simulink model "DAAEncounter"  (R2018b)
settings: Solver=ode45  StartTime=0.0  StopTime=180  RelTol=1e-3  EnableMultiTasking=on
values from neighbouring files (symbols this model uses):
  enableHorzMan = 1    [DAAEncounterClass.m]
  enableVertMan = 0    [DAAEncounterClass.m]
  eventFileNames = {'event1'; 'event2'}    [DAAEncounterClass.m]
  ignorePrevAlert = 1    [DAAEncounterClass.m]
  sim_sampleTime = 0.1    [DAAEncounterClass.m]
undefined symbols (not defined in the file or in its folder): daa_turnRate_dps, daa_vertRate_fpm, dh_flag, dh_ftps, dpsi_flag, dpsi_radps, uasPilot_altitudeK, uasPilot_altitudeOffset, uasPilot_altitudeTheta, uasPilot_coordDelayK, uasPilot_coordDelayMin, uasPilot_coordDelayTheta, uasPilot_desiredTurnRate_dps, uasPilot_desiredVertRate_ftpm, uasPilot_deterministicMode, uasPilot_dt_s, uasPilot_executionDelayMin, uasPilot_executionDelayMu, uasPilot_initialDelayMin, uasPilot_initialDelayMu, uasPilot_maxRelativeHdg, uasPilot_meanUpdateTimes, uasPilot_mentalFilter_climbThresh_fps, uasPilot_mentalFilter_numSamp, uasPilot_mentalFilter_turnThresh_rad, uasPilot_minUpdateTimes, uasPilot_operatorEnabled, uasPilot_probDescend, uasPilot_probFollowMinDev, uasPilot_probLeftTurn, uasPilot_probTurn, uasPilot_reducedClimbAlt_ft, uasPilot_reducedTurnAngle_deg, uasPilot_seedChoose, uasPilot_seedCoordDelay, uasPilot_seedExecutionDelay, uasPilot_seedInitialDelay, uasPilot_seedTurn, uasPilot_seedUpdate, uasPilot_seedVertical, uasPilot_triggerLevel, uasPilot_turnK, uasPilot_turnOffset, uasPilot_turnTheta
libraries: simulink x4, BasicAircraftDynamicsBlock x3, FlattenAircraftEstimateBus x2, PerfectSurveillanceBlock x2, DaidalusV201Block x1, HysteresisFilterBlock x1, MofNFilterBlock x1, CommonMetricsBlock x1, SLoWCBlock x1, WellClearMetricsBlock x1, NullAircraftEstimateBus x1, uas_pilot_model_r6 x1
(part 2 of 2)

== system DAAEncounter/Ownship Dynamics and Trajectory/Nominal Commands and Trajectory ==
  AC1 - Basic Aircraft Dynamics : BasicAircraftDynamicsBlock/Basic Aircraft Dynamics  ts_dynamics=.1  v_ftps_0=ac1dyn_v_ftps  N_ft_0=ac1dyn_N_ft  E_ft_0=ac1dyn_E_ft  h_ft_0=ac1dyn_h_ft  psi_rad_0=ac1dyn_psi_rad  theta_rad_0=ac1dyn_theta_rad  phi_rad_0=ac1dyn_phi_rad  a_ftpss_0=ac1dyn_a_ftpss  v_ftps_max=ac1dyn_con.maxAirspeed_ftps  v_ftps_min=ac1dyn_con.minAirspeed_ftps  dv_ftpss_max=ac1dyn_con.maxAcceleration_ftpss  dv_ftpss_min=ac1dyn_con.minAcceleration_ftpss  dh_ftps_max=ac1dyn_con.maxVerticalRate_ftps  dh_ftps_min=ac1dyn_con.minVerticalRate_ftps  q_radps_max=ac1dyn_con.maxPitchRate_radps  phi_rad_max=ac1dyn_con.maxBankAngle_rad  dphi_radps_max=ac1dyn_con.maxRollRate_radps  r_radps_max=ac1dyn_con.maxYawRate_radps  pNUM=ac1dyn_con.dynamicsNumeratorRollRate  pDEN=ac1dyn_con.dynamicsDenominatorRollRate  hNUM=ac1dyn_con.dynamicsNumeratorVerticalRate  hDEN=ac1dyn_con.dynamicsDenominatorVerticalRate  rNUM=ac1dyn_con.dynamicsNumeratorYawRate  rDEN=ac1dyn_con.dynamicsDenominatorYawRate  lat0_rad=ac2dyn_lat0_rad  lon0_rad=ac2dyn_lon0_rad  alt_ft=ac2dyn_alt0_ft
  AC1 - Nominal Trajectory : Subsystem  AncestorBlock=NominalTrajectory/Nominal Trajectory  mask(Logic and Response: Nominal Trajectory){eventFilename=eventFileNames{1}, ts=.1}
      mask prompts: eventFilename "Event matrix mat filename"; ts "Dynamic Update Rate"
      mask help:
      | The "Nominal Trajectory" Logic and Response Block describes the nominal
      | trajectory of an aircraft as defined in a "event matrix" typically sampled
      | from the encounter model.
      |
      | Logic and Response: Nominal Trajectory loads aircaft motion
      | commands from a MATLAB MAT file containing an event matrix of climb rates,
      | turn rates, and longitudinal accelerations, and presents them as a
      | CASSATT v6 AircraftCommands bus.
      |
      | The specified MAT file must contain a single matrix variable with four
      | rows.  The rows are
      |   - Time of control value change in seconds
      |   - Climb rate in feet per second
      |   - Turn rate in radians per second
      |   - Longitudinal acceleration in feet per second squared
      |
      | These control quantities (climb rate, turn rate acceleration) are assumed
      | remain constant between the times specified in the event matrix (zero order
      | hold).  The first / last control values in the event matrix are assumed to
      | preexist / persist at the value infinitely backwards / forwards in time.
      mask init:
      | set_param( [ gcb '/FromFile' ], 'Filename', eventFilename )
      mask Help:
      | The "Nominal Trajectory" Logic and Response Block describes the nominal
      | trajectory of an aircraft as defined in a "event matrix" typically sampled
      | from the encounter model.
      | 
      | Logic and Response: Nominal Trajectory loads aircaft motion
      | commands from a MATLAB MAT file containing an event matrix of climb rates,
      | turn rates, and longitudinal accelerations, and presents them as a
      | CASSATT v6 AircraftCommands bus.
      | 
      | The specified MAT file must contain a single matrix variable with four
      | rows.  The rows are
      |   - Time of control value change in seconds
      |   - Climb rate in feet per second
      |   - Turn rate in radians per second
      |   - Longitudinal acceleration in feet per second squared
      | 
      | These control quantities (climb rate, turn rate acceleration) are assumed
      | remain constant between the times specified in the event matrix (zero order
      | hold).  The first / last control values in the event matrix are assumed to
      | preexist / persist at the value infinitely backwards / forwards in time.
      | 
      | CASSATT v6 Aircraft dynamics blocks, which calculate the positions and velocities
      | traced out by an aircraft's trajectory,
      | require input signals specifying controls for the aircraft (e.g. turn rate, acceleration, climb rate)
      | in the form of a AircraftCommands bus.
      | This block allows the user to specify what these controls in a Matlab MAT file.
      | Include this in your simulation to describe the nominal motion of an aircraft
      | trajectory you have sampled from the Lincoln Encounter Models.
  Terminator : Terminator
  Nominal Commands : Outport
  NominalOwnshipState : Outport  Port=2
  NominalOwnshipStateRate : Outport  Port=3
  wires:
  AC1 - Nominal Trajectory/1(Aircraft Commands) -> AC1 - Basic Aircraft Dynamics/1, Nominal Commands/1
  AC1 - Basic Aircraft Dynamics/1 -> NominalOwnshipState/1  "Aircraft1"
  AC1 - Basic Aircraft Dynamics/2 -> Terminator/1
  AC1 - Basic Aircraft Dynamics/3 -> NominalOwnshipStateRate/1

== system DAAEncounter/Pilot/Format Maneuver As AircraftCommand ==
  Maneuver Flag : Inport  OutDataTypeStr=boolean
  Hrz Maneuver : Inport  Port=2
  Vrt Maneuver : Inport  Port=3
  Nominal Cmd : Inport  Port=4  OutDataTypeStr=Bus: AircraftCommands
  Own State : Inport  Port=5  OutDataTypeStr=Bus: AircraftState
  UAS Nominal Traj : Inport  Port=6
  Get Previous Command : Subsystem
  Horizontal Maneuver : Subsystem  TreatAsAtomicUnit=on
  Unit Delay : UnitDelay  SampleTime=-1
  Vertical Maneuver : Subsystem  TreatAsAtomicUnit=on
  Command Out : Outport  OutDataTypeStr=Bus: AircraftCommands
  wires:
  Maneuver Flag/1 -> Vertical Maneuver/4(Maneuver Flag), Horizontal Maneuver/4(Maneuver Flag), Get Previous Command/3(Maneuver Flag)
  Nominal Cmd/1 -> Get Previous Command/2(Nominal Cmd)
  Unit Delay/1 -> Get Previous Command/1(Cmd In)
  Own State/1 -> Vertical Maneuver/3(Own State), Horizontal Maneuver/3(Own State)
  Hrz Maneuver/1 -> Horizontal Maneuver/2(Maneuver)
  Vrt Maneuver/1 -> Vertical Maneuver/2(Maneuver)
  Horizontal Maneuver/1(Cmd Out) -> Vertical Maneuver/1(Command In)
  Vertical Maneuver/1(Cmd Out) -> Command Out/1, Unit Delay/1
  Get Previous Command/1(Cmd Out) -> Horizontal Maneuver/1(Command In)
  UAS Nominal Traj/1 -> Vertical Maneuver/5(UAS Nominal Traj)

== system DAAEncounter/Pilot/Horizontal and Vertical guidance enabler ==
  Unmodified Guidance : Inport
  " " : Constant  Value=enableVertMan
  " 1" : Constant  Value=enableHorzMan
  Horizontal Band manipulation : MATLAB Function  TreatAsAtomicUnit=on
  Switch : Switch  Criteria=u2 > Threshold
  Switch1 : Switch  Criteria=u2 > Threshold
  Vertical Band manipulation : MATLAB Function  TreatAsAtomicUnit=on
  Modified Guidance : Outport
  wires:
  " "/1 -> Switch/2
  Vertical Band manipulation/1(Guidance_out) -> Switch/3  "Guidance"
  Unmodified Guidance/1 -> Vertical Band manipulation/1(Guidance_in), Switch/1
  " 1"/1 -> Switch1/2
  Switch/1 -> Switch1/1, Horizontal Band manipulation/1(Guidance_in)
  Switch1/1 -> Modified Guidance/1
  Horizontal Band manipulation/1(Guidance_out) -> Switch1/3

== system DAAEncounter/Pilot/Subsystem ==
  Own State : Inport
  Alert Level : Inport  Port=2
  Trigger : Inport  Port=3
  Guidance : Inport  Port=4
  Max Turn Rt : Inport  Port=5
  Max Vert Rt : Inport  Port=6
  Enable : EnablePort
  Null AircraftEstimate Bus : NullAircraftEstimateBus/Null AircraftEstimate Bus
  UAS Pilot Model Release 6.1 : uas_pilot_model_r6/UAS Pilot Model Release 6.1  dt=dt  operator_enabled=operator_enabled  deterministicMode=deterministicMode  mean_initial_delay=mean_initial_delay  min_initial_delay=min_initial_delay  coord_delay_k=coord_delay_k  coord_delay_theta=coord_delay_theta  coord_delay_min=coord_delay_min  mean_exec_delay=mean_exec_delay  min_exec_delay=min_exec_delay  min_upd_times=min_upd_times  mean_upd_times=mean_upd_times  rng_seed_initial=rng_seed_initial  rng_seed_coord=rng_seed_coord  rng_seed_execution=rng_seed_execution  rng_seed_update=rng_seed_update  prob_follow_min=prob_follow_min  prob_turn_left=prob_turn_left  prob_turn_table=prob_turn  max_hdg_diff=max_hdg_diff  prob_descend=prob_descend  turn_k=turn_k  turn_theta=turn_theta  turn_offset=turn_offset  turn_k_alt=uasPilot_turnK_alt  turn_theta_alt=uasPilot_turnTheta_alt  turn_offset_alt=uasPilot_turnOffset_alt  alt_k=alt_k  alt_theta=alt_theta  alt_offset=alt_offset  rng_seed_horz=rng_seed_horz  rng_seed_vert=rng_seed_vert  rng_seed_horz_vs_vert=rng_seed_horz_vs_vert  mental_filter_samples=0  mental_filter_climb_thresh=0  mental_filter_turn_thresh=0
  Maneuver Flag : Outport
  Hrz Maneuver : Outport  Port=2
  Vrt Maneuver : Outport  Port=3
  wires:
  Own State/1 -> UAS Pilot Model Release 6.1/1
  Null AircraftEstimate Bus/1 -> UAS Pilot Model Release 6.1/2
  UAS Pilot Model Release 6.1/2 -> Hrz Maneuver/1
  Guidance/1 -> UAS Pilot Model Release 6.1/5
  Max Turn Rt/1 -> UAS Pilot Model Release 6.1/6
  Trigger/1 -> UAS Pilot Model Release 6.1/4
  Alert Level/1 -> UAS Pilot Model Release 6.1/3
  UAS Pilot Model Release 6.1/3 -> Vrt Maneuver/1
  UAS Pilot Model Release 6.1/1 -> Maneuver Flag/1
  Max Vert Rt/1 -> UAS Pilot Model Release 6.1/7

== system DAAEncounter/Pilot/Trigger ==
  Alert Level : Inport
  Filter Alerts : Subsystem  AncestorBlock=CABSAA_ModelLibrary/Filter Alerts  mask(Filter Alerts){trigger_level=trigger_level}
      mask prompts: trigger_level "Alert Level for Trigger"
      mask help: Holds alert level for at least the specified time unless the alert level increases.
  Trigger : Outport
  wires:
  Filter Alerts/1(Trigger) -> Trigger/1
  Alert Level/1 -> Filter Alerts/1(Alert Level In)

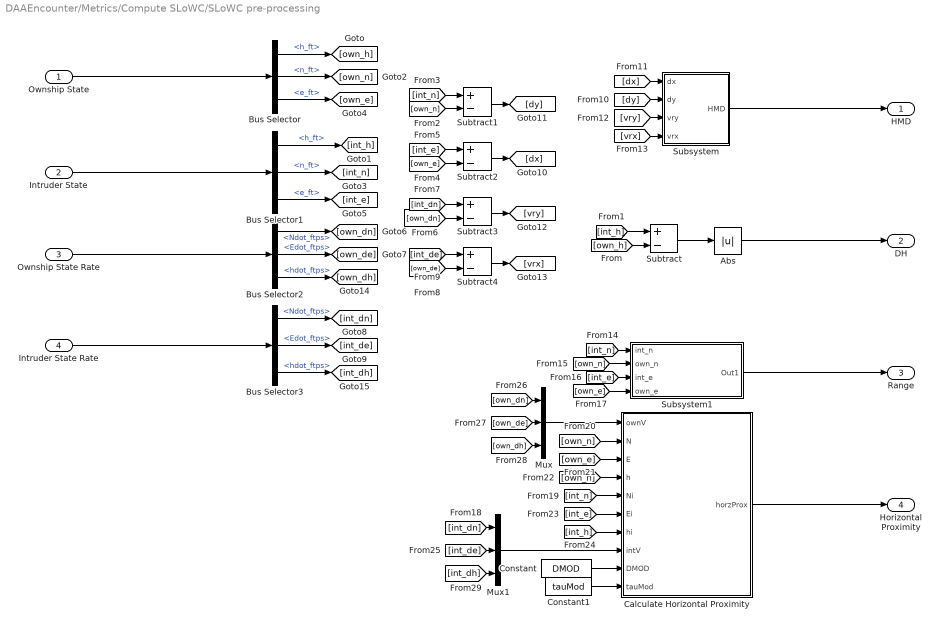
== system DAAEncounter/Metrics/Compute SLoWC/SLoWC pre-processing ==
  Ownship State : Inport
  Intruder State : Inport  Port=2
  Ownship State Rate : Inport  Port=3
  Intruder State Rate : Inport  Port=4
  Abs : Abs
  Bus Selector : BusSelector  OutputSignals=h_ft,n_ft,e_ft
  Bus Selector1 : BusSelector  OutputSignals=h_ft,n_ft,e_ft
  Bus Selector2 : BusSelector  OutputSignals=Ndot_ftps,Edot_ftps,hdot_ftps
  Bus Selector3 : BusSelector  OutputSignals=Ndot_ftps,Edot_ftps,hdot_ftps
  Calculate Horizontal Proximity : MATLAB Function  TreatAsAtomicUnit=on
  Constant : Constant  Value=DMOD
  Constant1 : Constant  Value=tauMod
  Mux : Mux  Inputs=3
  Mux1 : Mux  Inputs=3
  Subsystem : Subsystem
  Subsystem1 : Subsystem
  Subtract{,1..4} (5 alike) : Sum  Inputs=+-
  HMD : Outport
  DH : Outport  Port=2
  Range : Outport  Port=3
  Horizontal Proximity : Outport  Port=4
  wires:
  Subtract/1 -> Abs/1
  [own_dh] -> Mux/3
  Bus Selector/1 -> [own_h]  "<h_ft>"
  [own_dn] -> Subtract3/2
  Bus Selector1/3 -> [int_e]  "<e_ft>"
  [int_n] -> Calculate Horizontal Proximity/5(Ni)
  Bus Selector3/3 -> [int_dh]  "<hdot_ftps>"
  [int_h] -> Calculate Horizontal Proximity/7(hi)
  [int_e] -> Subtract2/1
  [own_h] -> Subtract/2
  Intruder State/1 -> Bus Selector1/1
  [own_n] -> Subtract1/2
  Constant/1 -> Calculate Horizontal Proximity/9(DMOD)
  [own_e] -> Subtract2/2
  [int_dh] -> Mux1/3
  Subtract4/1 -> [vrx]
  [int_h] -> Subtract/1
  Bus Selector1/1 -> [int_h]  "<h_ft>"
  [vry] -> Subsystem/3(vry)
  [own_n] -> Calculate Horizontal Proximity/2(N)
  Bus Selector3/1 -> [int_dn]  "<Ndot_ftps>"
  Subtract2/1 -> [dx]
  Bus Selector1/2 -> [int_n]  "<n_ft>"
  Bus Selector/2 -> [own_n]  "<n_ft>"
  Subtract3/1 -> [vry]
  [int_e] -> Subsystem1/3(int_e)
  [own_de] -> Mux/2
  Mux1/1 -> Calculate Horizontal Proximity/8(intV)
  Subtract1/1 -> [dy]
  [own_h] -> Calculate Horizontal Proximity/4(h)
  [dy] -> Subsystem/2(dy)
  [own_n] -> Subsystem1/2(own_n)
  [int_dn] -> Mux1/1
  Subsystem/1(HMD) -> HMD/1
  Bus Selector2/2 -> [own_de]  "<Edot_ftps>"
  [int_n] -> Subtract1/1
  Bus Selector2/3 -> [own_dh]  "<hdot_ftps>"
  [int_de] -> Subtract4/1
  Constant1/1 -> Calculate Horizontal Proximity/10(tauMod)
  Bus Selector/3 -> [own_e]  "<e_ft>"
  Subsystem1/1(Out1) -> Range/1
  [int_n] -> Subsystem1/1("int_n ")
  [int_e] -> Calculate Horizontal Proximity/6(Ei)
  [own_de] -> Subtract4/2
  Bus Selector3/2 -> [int_de]  "<Edot_ftps>"
  Mux/1 -> Calculate Horizontal Proximity/1(ownV)
  [dx] -> Subsystem/1("dx ")
  [int_dn] -> Subtract3/1
  Intruder State Rate/1 -> Bus Selector3/1
  [vrx] -> Subsystem/4(vrx)
  [own_dn] -> Mux/1
  Bus Selector2/1 -> [own_dn]  "<Ndot_ftps>"
  Abs/1 -> DH/1
  [own_e] -> Calculate Horizontal Proximity/3(E)
  Calculate Horizontal Proximity/1(horzProx) -> Horizontal Proximity/1
  Ownship State/1 -> Bus Selector/1
  [int_de] -> Mux1/2
  [own_e] -> Subsystem1/4(own_e)
  Ownship State Rate/1 -> Bus Selector2/1

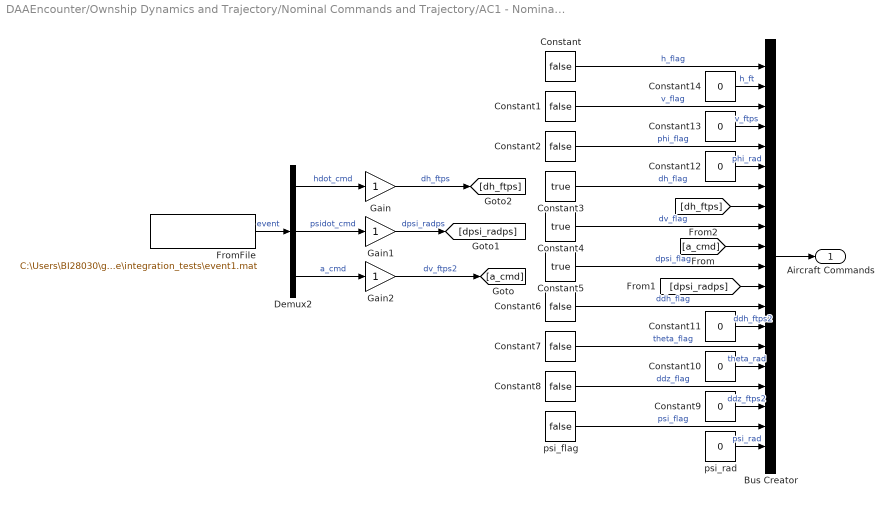
== system DAAEncounter/Ownship Dynamics and Trajectory/Nominal Commands and Trajectory/AC1 - Nominal Trajectory ==
  Bus Creator : BusCreator  Inputs=20  OutDataTypeStr=Bus: AircraftCommands  NonVirtualBus=on
  Constant{,1..2,6..8} (6 alike) : Constant  Value=false
  Constant{9..14} (6 alike) : Constant  Value=0
  Constant3 : Constant  Value=true
  Constant4 : Constant  Value=true
  Constant5 : Constant  Value=true
  Demux2 : Demux  Outputs=3
  FromFile : FromFile  FileName=C:\Users\BI28030\git_cln\DEGAS_cln\D_cln\CASSATT\code\integration_tests\event1.mat  SampleTime=ts  ExtrapolationBeforeFirstDataPoint=Hold first value  InterpolationWithinTimeRange=Zero order hold  ExtrapolationAfterLastDataPoint=Hold last value
  Gain : Gain
  Gain1 : Gain
  Gain2 : Gain
  psi_flag : Constant  Value=false
  psi_rad : Constant  Value=0
  Aircraft Commands : Outport  OutDataTypeStr=Bus: AircraftCommands
  wires:
  [dh_ftps] -> Bus Creator/8
  [dpsi_radps] -> Bus Creator/12
  [a_cmd] -> Bus Creator/10
  psi_rad/1 -> Bus Creator/20  "psi_rad"
  psi_flag/1 -> Bus Creator/19  "psi_flag"
  Demux2/1 -> Gain/1  "hdot_cmd"
  Demux2/2 -> Gain1/1  "psidot_cmd"
  Demux2/3 -> Gain2/1  "a_cmd"
  FromFile/1 -> Demux2/1  "event"
  Bus Creator/1 -> Aircraft Commands/1
  Constant/1 -> Bus Creator/1  "h_flag"
  Constant1/1 -> Bus Creator/3  "v_flag"
  Constant2/1 -> Bus Creator/5  "phi_flag"
  Constant3/1 -> Bus Creator/7  "dh_flag"
  Constant4/1 -> Bus Creator/9  "dv_flag"
  Constant5/1 -> Bus Creator/11  "dpsi_flag"
  Constant6/1 -> Bus Creator/13  "ddh_flag"
  Constant7/1 -> Bus Creator/15  "theta_flag"
  Constant8/1 -> Bus Creator/17  "ddz_flag"
  Gain/1 -> [dh_ftps]  "dh_ftps"
  Gain1/1 -> [dpsi_radps]  "dpsi_radps"
  Gain2/1 -> [a_cmd]  "dv_ftps2"
  Constant9/1 -> Bus Creator/18  "ddz_ftps2"
  Constant11/1 -> Bus Creator/14  "ddh_ftps2"
  Constant10/1 -> Bus Creator/16  "theta_rad"
  Constant14/1 -> Bus Creator/2  "h_ft"
  Constant13/1 -> Bus Creator/4  "v_ftps"
  Constant12/1 -> Bus Creator/6  "phi_rad"

== system DAAEncounter/Pilot/Format Maneuver As AircraftCommand/Get Previous Command ==
  Cmd In : Inport
  Nominal Cmd : Inport  Port=2
  Maneuver Flag : Inport  Port=3
  Data Type Conversion : DataTypeConversion  OutDataTypeStr=double
  Memory : Memory  InheritSampleTime=on
  Switch : Switch  Criteria=u2 > Threshold
  Cmd Out : Outport
  wires:
  Maneuver Flag/1 -> Memory/1
  Memory/1 -> Data Type Conversion/1
  Nominal Cmd/1 -> Switch/3
  Switch/1 -> Cmd Out/1
  Cmd In/1 -> Switch/1
  Data Type Conversion/1 -> Switch/2

== system DAAEncounter/Pilot/Format Maneuver As AircraftCommand/Horizontal Maneuver ==
  Command In : Inport
  Maneuver : Inport  Port=2
  Own State : Inport  Port=3
  Maneuver Flag : Inport  Port=4  OutDataTypeStr=boolean
  Bus Selector : BusSelector  OutputSignals=type
  Compare To Constant : simulink/Logic and Bit Operations/Compare To Constant  relop===  const=1  OutDataTypeStr=boolean
  Data Type Conversion1 : DataTypeConversion  OutDataTypeStr=double
  Logical Operator : Logic  AllPortsSameDT=off  OutDataTypeStr=boolean
  Set Desired Turn Rate : Subsystem
  Switch : Switch  Criteria=u2 > Threshold
  Cmd Out : Outport
  wires:
  Bus Selector/1 -> Compare To Constant/1  "<type>"
  Maneuver/1 -> Set Desired Turn Rate/2(Maneuver Magnitude), Bus Selector/1
  Own State/1 -> Set Desired Turn Rate/3(Own State)
  Maneuver Flag/1 -> Data Type Conversion1/1
  Logical Operator/1 -> Switch/2
  Command In/1 -> Switch/3, Set Desired Turn Rate/1(Cmd In)
  Data Type Conversion1/1 -> Logical Operator/1
  Compare To Constant/1 -> Logical Operator/2
  Set Desired Turn Rate/1(Cmd Out) -> Switch/1
  Switch/1 -> Cmd Out/1

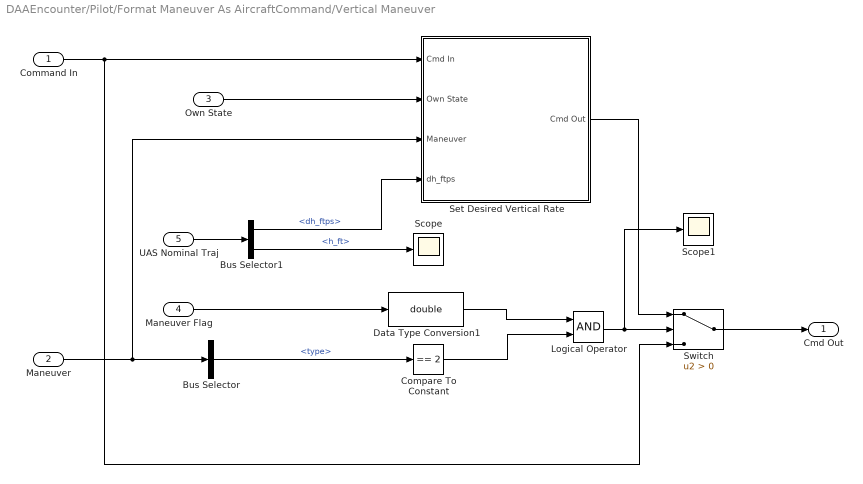
== system DAAEncounter/Pilot/Format Maneuver As AircraftCommand/Vertical Maneuver ==
  Command In : Inport
  Maneuver : Inport  Port=2
  Own State : Inport  Port=3
  Maneuver Flag : Inport  Port=4  OutDataTypeStr=boolean
  UAS Nominal Traj : Inport  Port=5
  Bus Selector1 : BusSelector  OutputSignals=dh_ftps,h_ft
  Bus Selector : BusSelector  OutputSignals=type
  Compare To Constant : simulink/Logic and Bit Operations/Compare To Constant  relop===  const=2  OutDataTypeStr=boolean
  Data Type Conversion1 : DataTypeConversion  OutDataTypeStr=double
  Logical Operator : Logic  AllPortsSameDT=off  OutDataTypeStr=boolean
  Scope : Scope
  Scope1 : Scope
  Set Desired Vertical Rate : Subsystem
  Switch : Switch  Criteria=u2 > Threshold
  Cmd Out : Outport
  wires:
  Bus Selector/1 -> Compare To Constant/1  "<type>"
  Maneuver Flag/1 -> Data Type Conversion1/1
  Switch/1 -> Cmd Out/1
  Data Type Conversion1/1 -> Logical Operator/1
  Compare To Constant/1 -> Logical Operator/2
  Command In/1 -> Set Desired Vertical Rate/1(Cmd In), Switch/3
  Set Desired Vertical Rate/1(Cmd Out) -> Switch/1
  UAS Nominal Traj/1 -> Bus Selector1/1
  Bus Selector1/2 -> Scope/1  "<h_ft>"
  Own State/1 -> Set Desired Vertical Rate/2(Own State)
  Maneuver/1 -> Set Desired Vertical Rate/3(Maneuver), Bus Selector/1
  Bus Selector1/1 -> Set Desired Vertical Rate/4(dh_ftps)  "<dh_ftps>"
  Logical Operator/1 -> Scope1/1, Switch/2

== system DAAEncounter/Pilot/Trigger/Filter Alerts ==
  Alert Level In : Inport
  Constant6 : Constant  Value=trigger_level
  Relational Operator : RelationalOperator  OutDataTypeStr=boolean  RndMeth=Nearest
  Trigger : Outport
  wires:
  Relational Operator/1 -> Trigger/1
  Constant6/1 -> Relational Operator/2
  Alert Level In/1 -> Relational Operator/1

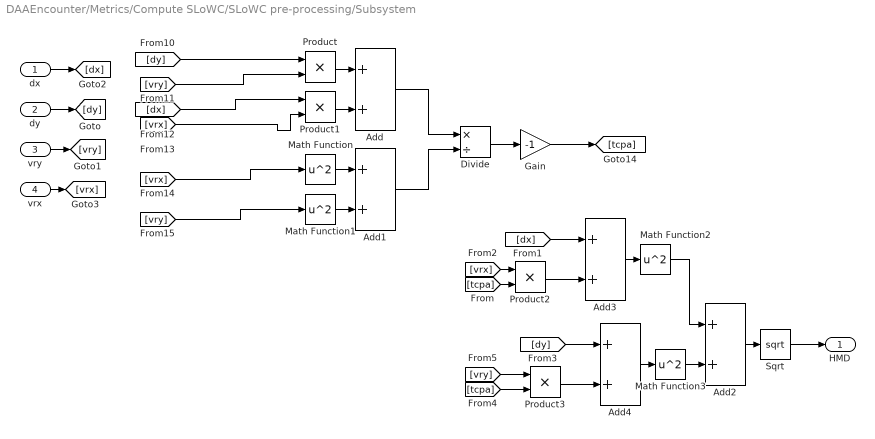
== system DAAEncounter/Metrics/Compute SLoWC/SLoWC pre-processing/Subsystem ==
  "dx " : Inport
  dy : Inport  Port=2
  vry : Inport  Port=3
  vrx : Inport  Port=4
  Add{,1..4} (5 alike) : Sum
  Divide : Product  Inputs=*/
  Gain : Gain  Gain=-1
  Math Function{,1..3} (4 alike) : Math  Operator=square  SaturateOnIntegerOverflow=on
  Product{,1..3} (4 alike) : Product
  Sqrt : Sqrt  SaturateOnIntegerOverflow=on
  HMD : Outport
  wires:
  Math Function1/1 -> Add1/2
  Gain/1 -> [tcpa]
  Add/1 -> Divide/1
  Math Function/1 -> Add1/1
  Product1/1 -> Add/2
  Product/1 -> Add/1
  [vrx] -> Math Function/1
  [vrx] -> Product1/2
  [dx] -> Product1/1
  Divide/1 -> Gain/1
  Add1/1 -> Divide/2
  [vry] -> Product/2
  [dy] -> Product/1
  [vry] -> Math Function1/1
  Sqrt/1 -> HMD/1
  Add2/1 -> Sqrt/1
  Math Function2/1 -> Add2/1
  Add3/1 -> Math Function2/1
  [dx] -> Add3/1
  [vrx] -> Product2/1
  Product2/1 -> Add3/2
  [tcpa] -> Product2/2
  Add4/1 -> Math Function3/1
  Math Function3/1 -> Add2/2
  Product3/1 -> Add4/2
  [dy] -> Add4/1
  [tcpa] -> Product3/2
  [vry] -> Product3/1
  "dx "/1 -> [dx]
  vrx/1 -> [vrx]
  vry/1 -> [vry]
  dy/1 -> [dy]

== system DAAEncounter/Metrics/Compute SLoWC/SLoWC pre-processing/Subsystem1 ==
  "int_n " : Inport
  own_n : Inport  Port=2
  int_e : Inport  Port=3
  own_e : Inport  Port=4
  Add1 : Sum
  Math Function : Math  Operator=square  SaturateOnIntegerOverflow=on
  Math Function1 : Math  Operator=square  SaturateOnIntegerOverflow=on
  Sqrt : Sqrt  SaturateOnIntegerOverflow=on
  Subtract5 : Sum  Inputs=+-
  Subtract6 : Sum  Inputs=+-
  Out1 : Outport
  wires:
  Math Function/1 -> Add1/1
  Add1/1 -> Sqrt/1
  Math Function1/1 -> Add1/2
  Subtract5/1 -> Math Function/1
  Sqrt/1 -> Out1/1
  Subtract6/1 -> Math Function1/1
  int_e/1 -> Subtract6/1
  own_n/1 -> Subtract5/2
  "int_n "/1 -> Subtract5/1
  own_e/1 -> Subtract6/2

== system DAAEncounter/Pilot/Format Maneuver As AircraftCommand/Horizontal Maneuver/Set Desired Turn Rate ==
  Cmd In : Inport
  Maneuver Magnitude : Inport  Port=2
  Own State : Inport  Port=3
  Bus Assignment1 : BusAssignment  AssignedSignals=dpsi_flag,dpsi_radps
  Constant : Constant  OutDataTypeStr=boolean
  Desired Heading to Turn Rate : Subsystem
  Cmd Out : Outport
  wires:
  Own State/1 -> Desired Heading to Turn Rate/2(Own State)
  Bus Assignment1/1 -> Cmd Out/1
  Cmd In/1 -> Bus Assignment1/1
  Constant/1 -> Bus Assignment1/2
  Maneuver Magnitude/1 -> Desired Heading to Turn Rate/1(Heading Cmd)
  Desired Heading to Turn Rate/1(Turn Rate) -> Bus Assignment1/3

== system DAAEncounter/Pilot/Format Maneuver As AircraftCommand/Vertical Maneuver/Set Desired Vertical Rate ==
  Cmd In : Inport
  Own State : Inport  Port=2
  Maneuver : Inport  Port=3
  dh_ftps : Inport  Port=4
  Bus Assignment : BusAssignment  AssignedSignals=dh_flag,dh_ftps
  Constant : Constant  OutDataTypeStr=boolean
  Constant1 : Constant  Value=enableVertMan
  Desired Altitude to Vertical Rate : Subsystem
  Multiport Switch : MultiPortSwitch  DataPortOrder=Specify indices  DataPortIndices={1 0}
  Scope : Scope
  Cmd Out : Outport
  wires:
  Bus Assignment/1 -> Cmd Out/1
  Own State/1 -> Desired Altitude to Vertical Rate/2(Own State)
  Cmd In/1 -> Bus Assignment/1
  Constant/1 -> Bus Assignment/2
  Maneuver/1 -> Desired Altitude to Vertical Rate/1(Altitude Cmd)
  dh_ftps/1 -> Multiport Switch/3
  Constant1/1 -> Multiport Switch/1
  Desired Altitude to Vertical Rate/1(Vert Rt) -> Scope/1, Multiport Switch/2
  Multiport Switch/1 -> Bus Assignment/3

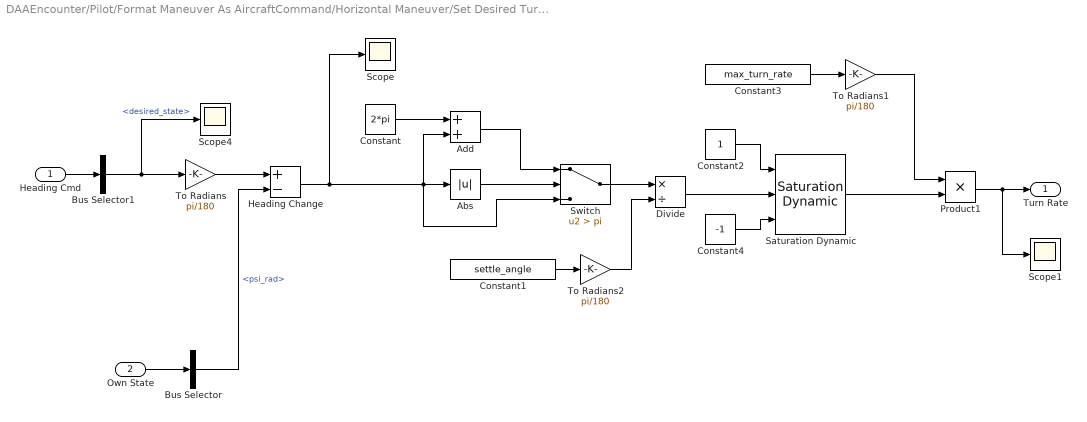
== system DAAEncounter/Pilot/Format Maneuver As AircraftCommand/Horizontal Maneuver/Set Desired Turn Rate/Desired Heading to Turn Rate ==
  Heading Cmd : Inport
  Own State : Inport  Port=2
  Abs : Abs
  Add : Sum
  Bus Selector : BusSelector  OutputSignals=psi_rad
  Bus Selector1 : BusSelector  OutputSignals=desired_state
  Constant : Constant  Value=2*pi
  Constant1 : Constant  Value=settle_angle
  Constant2 : Constant
  Constant3 : Constant  Value=max_turn_rate
  Constant4 : Constant  Value=-1
  Divide : Product  Inputs=*/
  Heading Change : Sum  Inputs=+-
  Product1 : Product  RndMeth=Zero
  Saturation Dynamic : simulink/Discontinuities/Saturation Dynamic  OutMin=[]  OutMax=[]  OutDataTypeStr=Inherit: Same as second input  OutDataType=fixdt(1, 16)  OutScaling=2^-10  DoSatur=off
  Scope : Scope
  Scope1 : Scope
  Scope4 : Scope
  Switch : Switch  Criteria=u2 > Threshold  Threshold=pi
  To Radians : Gain  Gain=pi/180
  To Radians1 : Gain  Gain=pi/180
  To Radians2 : Gain  Gain=pi/180
  Turn Rate : Outport
  wires:
  Constant/1 -> Add/1
  Switch/1 -> Divide/1
  Constant4/1 -> Saturation Dynamic/3
  Divide/1 -> Saturation Dynamic/2
  Abs/1 -> Switch/2
  Heading Change/1 -> Scope/1, Switch/3, Abs/1, Add/2
  Add/1 -> Switch/1
  Own State/1 -> Bus Selector/1
  Bus Selector/1 -> Heading Change/2  "<psi_rad>"
  To Radians/1 -> Heading Change/1
  Constant2/1 -> Saturation Dynamic/1
  Saturation Dynamic/1 -> Product1/2
  Constant1/1 -> To Radians2/1
  Product1/1 -> Scope1/1, Turn Rate/1
  Constant3/1 -> To Radians1/1
  To Radians1/1 -> Product1/1
  To Radians2/1 -> Divide/2
  Bus Selector1/1 -> To Radians/1, Scope4/1  "<desired_state>"
  Heading Cmd/1 -> Bus Selector1/1

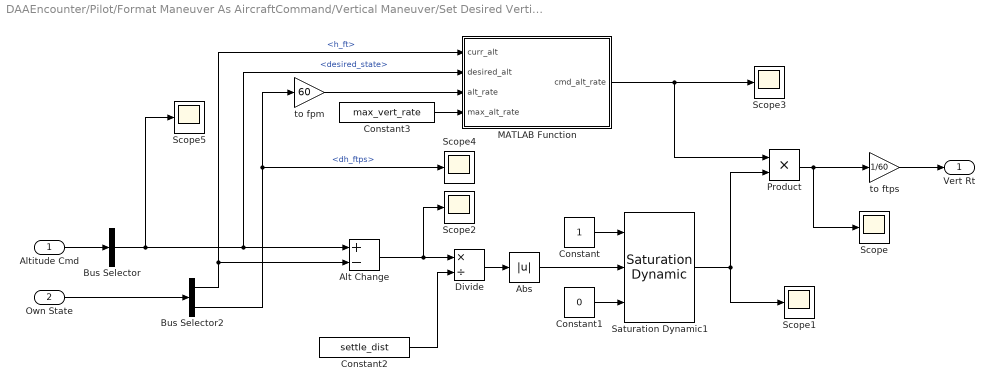
== system DAAEncounter/Pilot/Format Maneuver As AircraftCommand/Vertical Maneuver/Set Desired Vertical Rate/Desired Altitude to Vertical Rate ==
  Altitude Cmd : Inport
  Own State : Inport  Port=2
  Abs : Abs
  Alt Change : Sum  Inputs=+-
  Bus Selector : BusSelector  OutputSignals=desired_state
  Bus Selector2 : BusSelector  OutputSignals=h_ft,dh_ftps
  Constant : Constant
  Constant1 : Constant  Value=0
  Constant2 : Constant  Value=settle_dist
  Constant3 : Constant  Value=max_vert_rate
  Divide : Product  Inputs=*/
  MATLAB Function : MATLAB Function  TreatAsAtomicUnit=on
  Product : Product  RndMeth=Zero
  Saturation Dynamic1 : simulink/Discontinuities/Saturation Dynamic  OutMin=[]  OutMax=[]  OutDataTypeStr=Inherit: Same as second input  OutDataType=fixdt(1, 16)  OutScaling=2^-10  DoSatur=off
  Scope{,1..5} (6 alike) : Scope
  to fpm : Gain  Gain=60
  to ftps : Gain  Gain=1/60
  Vert Rt : Outport
  wires:
  Constant2/1 -> Divide/2
  Alt Change/1 -> Divide/1, Scope2/1
  Product/1 -> to ftps/1, Scope/1
  Own State/1 -> Bus Selector2/1
  Altitude Cmd/1 -> Bus Selector/1
  Bus Selector2/1 -> MATLAB Function/1(curr_alt), Alt Change/2  "<h_ft>"
  Divide/1 -> Abs/1
  Constant/1 -> Saturation Dynamic1/1
  Constant1/1 -> Saturation Dynamic1/3
  Saturation Dynamic1/1 -> Scope1/1, Product/2
  Abs/1 -> Saturation Dynamic1/2
  to ftps/1 -> Vert Rt/1
  Bus Selector/1 -> Scope5/1, MATLAB Function/2(desired_alt), Alt Change/1  "<desired_state>"
  Constant3/1 -> MATLAB Function/4(max_alt_rate)
  Bus Selector2/2 -> Scope4/1, to fpm/1  "<dh_ftps>"
  MATLAB Function/1(cmd_alt_rate) -> Scope3/1, Product/1
  to fpm/1 -> MATLAB Function/3(alt_rate)

== matlab function DAAEncounter/Pilot/Horizontal and Vertical guidance enabler/Vertical Band manipulation ==
  data: Guidance_in input; Guidance_out output
function Guidance_out = fcn(Guidance_in)

temp = Guidance_in;
temp(273) = 4;
temp(275) = 4;
temp(277) = 4;
temp(279) = 4;
temp(281) = 4;
temp(283) = 4;

Guidance_out = temp;

== matlab function DAAEncounter/Pilot/Horizontal and Vertical guidance enabler/Horizontal Band manipulation ==
  data: Guidance_in input; Guidance_out output
function Guidance_out = fcn(Guidance_in)

temp = Guidance_in;
temp(1:271) = 4;

Guidance_out = temp;

== matlab function DAAEncounter/Pilot/Format Maneuver As AircraftCommand/Vertical Maneuver/Set Desired Vertical Rate/Desired Altitude to Vertical Rate/MATLAB Function ==
  data: curr_alt input; cmd_alt_rate output; desired_alt input; alt_rate input; max_alt_rate input
function cmd_alt_rate = fcn(curr_alt, desired_alt, alt_rate, max_alt_rate)
%#codegen

if desired_alt >= curr_alt
  cmd_alt_rate = max_alt_rate;
else
  cmd_alt_rate = -max_alt_rate;
end

% override specified vertical rate for maneuvers if already climbing or
% descending in direction of desired altitude

% currently climbing
% if alt_rate > 0
%   
%   if desired_alt > curr_alt
%     cmd_alt_rate = alt_rate;
%   end
%   
% % currently descending
% elseif alt_rate < 0
%   
%   if desired_alt < curr_alt
%     cmd_alt_rate = alt_rate;
%   end
%   
% end

== matlab function DAAEncounter/Metrics/Compute SLoWC/SLoWC pre-processing/Calculate Horizontal Proximity ==
  data: ownV input; N input; horzProx output; E input; h input; Ni input; Ei input; hi input; intV input; DMOD input; tauMod input
function horzProx = getHorzProx(ownV,N,E,h,Ni,Ei,hi,intV, DMOD, tauMod) 
% This block computes horizontal proximity (S_i in the Bihrle slide 3)

%Ri = [Ni-N; Ei-E; -(hi-h)];
Ri = [Ni-N; Ei-E; 0];

rangeRate = 0;

if(~isempty(Ri) && ~isempty(ownV) && ~isempty(intV))
    relVel = intV - ownV;
    rangeRate = dot(Ri/norm(Ri), relVel);
end

horzProx = max(DMOD, 0.5* (sqrt((rangeRate*tauMod)^2 + 4*DMOD^2) - rangeRate*tauMod) );
